simulink model "ex1"  (R2017b)
settings: Solver=VariableStepAuto  StartTime=0.0  StopTime=10.0  RelTol=1e-3
settings Model: Creator=User  LastModifiedBy=User

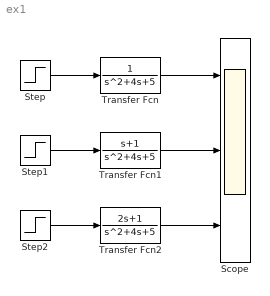
== system ex1 ==
  Scope : Scope  NumInputPorts=3
  Step : Step  Time=0  SampleTime=0
  Step1 : Step  Time=0  SampleTime=0
  Step2 : Step  Time=0  SampleTime=0
  Transfer Fcn : TransferFcn  Denominator=[1 4 5]
  Transfer Fcn1 : TransferFcn  Numerator=[1 1]  Denominator=[1 4 5]
  Transfer Fcn2 : TransferFcn  Numerator=[2 1]  Denominator=[1 4 5]
  wires:
  Step/1 -> Transfer Fcn/1
  Step1/1 -> Transfer Fcn1/1
  Step2/1 -> Transfer Fcn2/1
  Transfer Fcn/1 -> Scope/1
  Transfer Fcn1/1 -> Scope/2
  Transfer Fcn2/1 -> Scope/3
